simulink model "hireAdnFireV1"  (R2016b)
settings: Solver=ode4  StartTime=0.0  StopTime=100.0  FixedStep=0.01  RelTol=1e-3
settings Model: Creator=Thomas  LastModifiedBy=Thomas

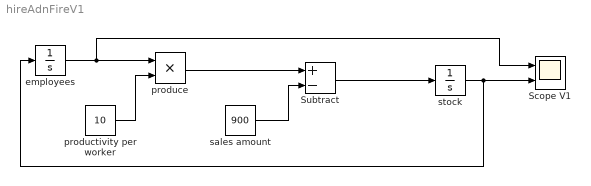
== system hireAdnFireV1 ==
  Scope V1 : Scope  NumInputPorts=2
  Subtract : Sum  Inputs=+-
  employees : Integrator  InitialCondition=50
  produce : Product
  productivity per worker : Constant  Value=10
  sales amount : Constant  Value=900
  stock : Integrator  InitialCondition=100
  wires:
  productivity per worker/1 -> produce/2
  stock/1 -> employees/1, Scope V1/2
  sales amount/1 -> Subtract/2
  Subtract/1 -> stock/1
  employees/1 -> Scope V1/1, produce/1
  produce/1 -> Subtract/1
